simulink model "full_state_linear_SPMSG"  (R2020b)
settings: Solver=FixedStepAuto  StartTime=0  StopTime=2  FixedStep=5e-7  RelTol=1e-3
undefined symbols (not defined in the file): capacitance, DiscIntNeverNeededParam, LdRated, LqRated, PhiPMRated, Pn, Rsnubber, RsRated, speed, TsimCurLoop, TsimMotor
libraries: powerlib x18, slpidlib x3, simulink x2, powerlib_meascontrol x2
(part 2 of 2)

== matlab function full_state_linear_SPMSG/motor/VSINonlinearity/MATLAB Function3 ==
  data: I input; U output; K input; Vdead input
function U = VSI_Nonlinearity(I,K,Vdead)
    U = Vdead*atan(I)/pi*2;
end

== matlab function full_state_linear_SPMSG/converter/800 ==
  data: y output
function y = fcn()
persistent t
if isempty(t)
    t=0;
end
t = t + 1;
if (t > 2.5e6)
    y = 45;
elseif (t > 1.5e6)
    y = 500;
else
    y = 45;
end

== matlab function full_state_linear_SPMSG/control algorithm/Subsystem1/system reconstruction ==
  settings: updateMethod=DISCRETE
  data: x1 input; z1 output; x2 input; x3 input; speed input; Lq_norm input; Ld_norm input; Cdc_norm input; Rs_norm input; Phi_dm_norm input; v1_in input; v2_in input; Rdc input; z2 output; z3 output; u1 output; u2 output; A output; E output; Rdc_est input
function [z1,z2,z3,u1,u2,A,E] = fcn(x1, x2, x3, speed, Lq_norm, Ld_norm, Cdc_norm, Rs_norm, Phi_dm_norm, v1_in, v2_in,Rdc, Rdc_est)
we = abs(speed)*2*pi/60*4+0.01;
z1 = 3/2*Lq_norm*x1*x1 + 3/2*Ld_norm*x2*x2 + Cdc_norm*x3;
z2 = -3*Rs_norm*(x1*x1+x2*x2) - 3*we*(Ld_norm-Lq_norm)*x1*x2 - 3*we*Phi_dm_norm*x1 - 2/Rdc_est*x3;
z3 = x2;
%inputs
v1 = v1_in;
v2 = v2_in;
V = [v1;v2];
%state transformation
f1 = -Rs_norm/Lq_norm*x1 - we*Ld_norm/Lq_norm*x2 - we*Phi_dm_norm/Lq_norm;
f2 = -Rs_norm/Ld_norm*x2 + we*Lq_norm/Ld_norm*x1;
f3 = -2/Cdc_norm/Rdc*x3;
f = [f1 f2 f3];
g1 = [1/Lq_norm 0 -3/Cdc_norm*x1];
g2 = [0 1/Ld_norm -3/Cdc_norm*x2];
Jacob_LfS11 = [-6*Rs_norm*x1-3*we*(Ld_norm-Lq_norm)*x2-3*we*Phi_dm_norm;
    -6*Rs_norm*x2-3*we*(Ld_norm-Lq_norm)*x1;
    -2/Rdc
    ];
Jacob_S21 = [0;
    1;
    0
    ];
LfLfS11 = f*Jacob_LfS11;
Lg1LfS11 = g1*Jacob_LfS11;
Lg2LfS11 = g2*Jacob_LfS11;
LfS21 = f*Jacob_S21;
Lg1S21 = g1*Jacob_S21;
Lg2S21 = g2*Jacob_S21;
E = 1e-4*[Lg1LfS11 Lg2LfS11;Lg1S21 Lg2S21];
A = [LfLfS11;LfS21];
U = E^-1*(-1e-4*A+V);
u1 = U(1);
u2 = U(2);

== matlab function full_state_linear_SPMSG/MATLAB Function ==
  data: Clock input
  events: INT_ENABLE output FUNCTION_CALL_EVENT
function SYS_ENABLE(Clock)
    if(Clock == 0)
        INT_ENABLE();
    end
end

== matlab function full_state_linear_SPMSG/control algorithm/Subsystem1/reference counting ==
  settings: updateMethod=DISCRETE
  data: iq output; udc_dem input; y output; Rdc input; speed input; Rs_norm input; Phi_dm_norm input; Lq_norm input; Cdc_norm input
function [iq,y] = fcn(udc_dem,Rdc, speed, Rs_norm, Phi_dm_norm, Lq_norm, Cdc_norm)
we = speed*2*pi/60*4;
a = Rs_norm;
b = we*Phi_dm_norm;
c = 2/3*udc_dem*udc_dem/Rdc;
iq = (-b+sqrt(abs(b*b-4*a*c)))/2/a;
y = 3*Lq_norm*iq*iq/2+Cdc_norm*udc_dem*udc_dem;

== matlab function full_state_linear_SPMSG/control algorithm/Subsystem1/MATLAB Function ==
  data: y output
function y = fcn()
persistent t
if isempty(t)
    t=0;
end
t = t + 1;
if (t > 50)
    y = 1;
else
    y = 0;
end

== matlab function full_state_linear_SPMSG/converter/1200 ==
  data: y output
function y = fcn()
persistent t
if isempty(t)
    t=0;
end
t = t + 1;
if (t > 2.5e6)
    y = 10;
elseif (t > 1.5e6)
    y = 20;
else
    y = 10;
end

== matlab function full_state_linear_SPMSG/control algorithm/SVPWM1/MATLAB Function1 ==
  data: alpha input; ta output; beta input; tb output; tc output
function [ta,tb,tc] = SVPWM(alpha,beta)

temp1=beta;
temp2=0.5*beta+0.86603*alpha;
temp3=temp2-temp1;

VecSector=3;
if(temp2>0)
    VecSector=VecSector-1;
end
if(temp3>0)
    VecSector=VecSector-1;
end
if(temp1<0)
    VecSector=7-VecSector;
end

switch VecSector
    case 1
        ta=temp2;
        tb=temp1-temp3;
        tc=-temp2;
    case 2
        ta=temp3+temp2;
        tb=temp1;
        tc=-temp1;
    case 3
        ta=temp3;
        tb=-temp3;
        tc=-(temp1+temp2);
    case 4
        ta=temp2;
        tb=temp1-temp3;
        tc=-temp2;
    case 5
        ta=temp3+temp2;
        tb=temp1;
        tc=-temp1;
    case 6
        ta=temp3;
        tb=-temp3;
        tc=-(temp1+temp2);
    otherwise
        ta=(0.5);
        tb=(0.5);
        tc=(0.5);
end

== matlab function full_state_linear_SPMSG/converter/1000 ==
  data: y output
function y = fcn()
persistent t
if isempty(t)
    t=0;
end
t = t + 1;
if (t > 2.5e6)
    y = 15;
elseif (t > 1.5e6)
    y = 40;
else
    y = 15;
end
